simulink model "myModel"  (R2013b)
settings: Solver=ode45  StartTime=0.0  StopTime=10.0  RelTol=1e-3
settings Model: Creator=Eduardo  LastModifiedBy=Eduardo
settings SFSimCC: SimCustomHeaderCode="#include \"doubleIt.h\""  SimUserSources=doubleIt.c

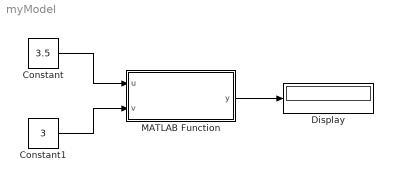
== system myModel ==
  Constant : Constant  Value=3.5
  Constant1 : Constant  Value=3
  Display : Display
  MATLAB Function : MATLAB Function  TreatAsAtomicUnit=on
  wires:
  Constant/1 -> MATLAB Function/1(u)
  MATLAB Function/1(y) -> Display/1
  Constant1/1 -> MATLAB Function/2(v)

== matlab function myModel/MATLAB Function ==
  data: u input; y output; v input
function y = callingDoubleIt(u, v)

y = 0.0;
y = coder.ceval('doubleIt',u, v);
